simulink model "untitled2"  (R2023b)
settings: Solver=VariableStepAuto  StartTime=0.0  StopTime=50  RelTol=1e-3
values from neighbouring files (symbols this model uses):
  b1 = 350    [untitled10.m]    (also in untitled4.m; untitled5.m)
  b2 = 15020    [untitled10.m]    (also in untitled4.m; untitled5.m)
  k1 = 80000    [untitled10.m]    (also in untitled4.m; untitled5.m)
  k2 = 500000    [untitled10.m]    (also in untitled4.m; untitled5.m)
  m1 = 2500    [untitled10.m]    (also in untitled4.m; untitled5.m)
  m2 = 320    [untitled10.m]    (also in untitled4.m; untitled5.m)
settings Model: Creator=youss  LastModifiedBy=youss

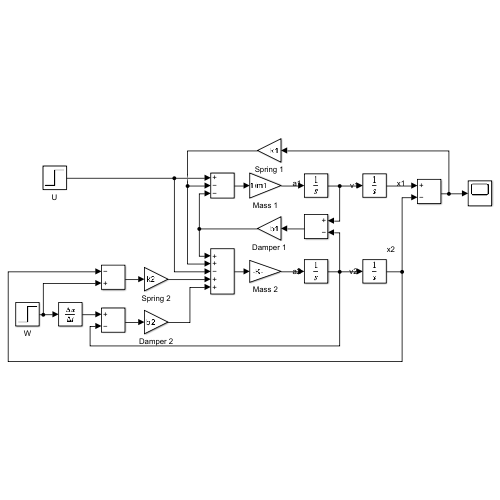
[thumbnail: Simulink's stored preview of the top-level diagram]
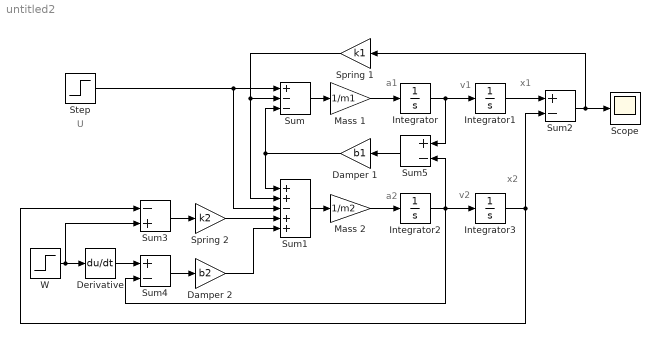
== system untitled2 ==
  note: U
  note: x1
  note: a1
  note: x2
  note: a2
  note: v1
  note: v2
  Damper 1 : Gain  Gain=b1  SaturateOnIntegerOverflow=on  OutDataTypeStr=Inherit: Same as input  ParamDataTypeStr=Inherit: Same as input
  Damper 2 : Gain  Gain=b2  SaturateOnIntegerOverflow=on  OutDataTypeStr=Inherit: Same as input  ParamDataTypeStr=Inherit: Same as input
  Derivative : Derivative
  Integrator{,1..3} (4 alike) : Integrator
  Mass 1 : Gain  Gain=1/m1  SaturateOnIntegerOverflow=on  OutDataTypeStr=Inherit: Same as input  ParamDataTypeStr=Inherit: Same as input
  Mass 2 : Gain  Gain=1/m2  SaturateOnIntegerOverflow=on  OutDataTypeStr=Inherit: Same as input  ParamDataTypeStr=Inherit: Same as input
  Scope : Scope
  Spring 1 : Gain  Gain=k1  SaturateOnIntegerOverflow=on  OutDataTypeStr=Inherit: Same as input  ParamDataTypeStr=Inherit: Same as input
  Spring 2 : Gain  Gain=k2  SaturateOnIntegerOverflow=on  OutDataTypeStr=Inherit: Same as input  ParamDataTypeStr=Inherit: Same as input
  Step : Step  Time=0  SampleTime=0
  Sum : Sum  Inputs=+--  InputSameDT=on  SaturateOnIntegerOverflow=on  OutDataTypeStr=Inherit: Same as first input
  Sum1 : Sum  Inputs=++-++  InputSameDT=on  SaturateOnIntegerOverflow=on  OutDataTypeStr=Inherit: Same as first input
  Sum2 : Sum  Inputs=+-  InputSameDT=on  SaturateOnIntegerOverflow=on  OutDataTypeStr=Inherit: Same as first input
  Sum3 : Sum  Inputs=-+  InputSameDT=on  SaturateOnIntegerOverflow=on  OutDataTypeStr=Inherit: Same as first input
  Sum4 : Sum  Inputs=+-  InputSameDT=on  SaturateOnIntegerOverflow=on  OutDataTypeStr=Inherit: Same as first input
  Sum5 : Sum  Inputs=+-  InputSameDT=on  SaturateOnIntegerOverflow=on  OutDataTypeStr=Inherit: Same as first input
  W : Step  Time=0  After=0
  wires:
  Step/1 -> Sum/1, Sum1/3
  Sum1/1 -> Mass 2/1
  Mass 1/1 -> Integrator/1
  Sum/1 -> Mass 1/1
  Mass 2/1 -> Integrator2/1
  Integrator2/1 -> Integrator3/1, Sum4/2, Sum5/2
  Spring 2/1 -> Sum1/4
  Derivative/1 -> Sum4/1
  W/1 -> Sum3/2, Derivative/1
  Sum3/1 -> Spring 2/1
  Integrator3/1 -> Sum2/2, Sum3/1
  Integrator/1 -> Integrator1/1, Sum5/1
  Spring 1/1 -> Sum/2, Sum1/2
  Damper 1/1 -> Sum1/1, Sum/3
  Sum5/1 -> Damper 1/1
  Integrator1/1 -> Sum2/1
  Damper 2/1 -> Sum1/5
  Sum2/1 -> Scope/1, Spring 1/1
  Sum4/1 -> Damper 2/1
